simulink model "nounity"  (R2020a)
settings: Solver=FixedStepAuto  StartTime=0.0  StopTime=200  FixedStep=.005  RelTol=1e-3
undefined symbols (not defined in the file or in its folder): dMaxX, dMaxY, dMinX, dMinY, dSeedX, dSeedY, dts, waPhi, waPsi, waTheta, waX, waY, waZ, wfPhi, wfPsi, wfTheta, wfX, wfY, wfZ, wpPhi, wpPsi, wpTheta, wpX, wpY, wpZ
libraries: sharedutil x1
settings Model: Creator=Lamarre  LastModifiedBy=Lamarre

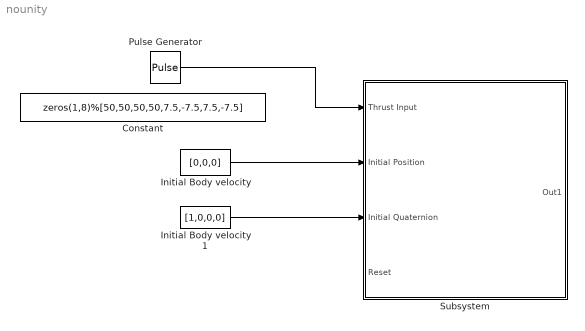
== system nounity ==
  Constant : Constant  Value=zeros(1,8)%[50,50,50,50,7.5,-7.5,7.5,-7.5]
  "Initial Body velocity " : Constant  Value=[0,0,0]
  Initial Body velocity 1 : Constant  Value=[1,0,0,0]
  Pulse Generator : DiscretePulseGenerator  PulseType=Time based  Amplitude=20  Period=10  PulseWidth=50
  Subsystem : Subsystem  InitFcn=|
      | % Initialiser le seed du random
      | rng shuffle
      | 
      | % Retrouver le paramètre de AUV8
      | cf = ConfigAUV8();
      | 
      | % Constante pour bloc areospace
      | %     I=cf.I;
      | %     mass=cf.mass;
      | 
      | % Perturbations des vages
      |     %Vages X
      |     waX=2;          % Amplitude
      |     wfX=pi/2;         % Frequence
      |     wpX=0;          % Phase
      |     %Vages Y
      |     waY=3;          % Amplitude
      |     wfY=pi/2;         % Frequence
      |     wpY=pi/2;       % Phase
      |     %Vages Z
      |     waZ= 4;         % Amplitude
      |     wfZ=pi/2;         % Frequence
      |     wpZ=pi;         % Phase
      |     %Vages RX (Roll)
      |     waPhi= 3;      % Amplitude
      |     wfPhi= pi/2;      % Frequence
      |     wpPhi=0;        % Phase
      |     %Vages Ry (Pitch)
      |     waTheta=3;    % Amplitude
      |     wfTheta=pi/2;     % Frequence
      |     wpTheta=pi/2;   % Phase
      |     %Vages Rz (Yaw)
      |     waPsi=3;       % Amplitude
      |     wfPsi=pi/2;       % Frequence
      |     wpPsi=pi;       % Phase
      |     
      | % Perturbation Drift
      | 
      |     dts=5; % Temp d'échantillionage des perturbation
      |     
      |     % Perturbation x
      |     dMinX=-1*rand(); % Valeur minimum x
      |     dMaxX=1*rand();  % Valeur maximum x
      |     dSeedX=round(rand*10);
      |     
      |     % Perturbation y
      |     dMinY=-3*rand(); % Valeur minimum  y
      |     dMaxY=3*rand();  % Valeur maximumx y
      |     dSeedY=round(rand*10);
  wires:
  "Initial Body velocity "/1 -> Subsystem/2(Initial Position)
  Initial Body velocity 1/1 -> Subsystem/3(Initial Quaternion)
  Pulse Generator/1 -> Subsystem/1(Thrust Input)

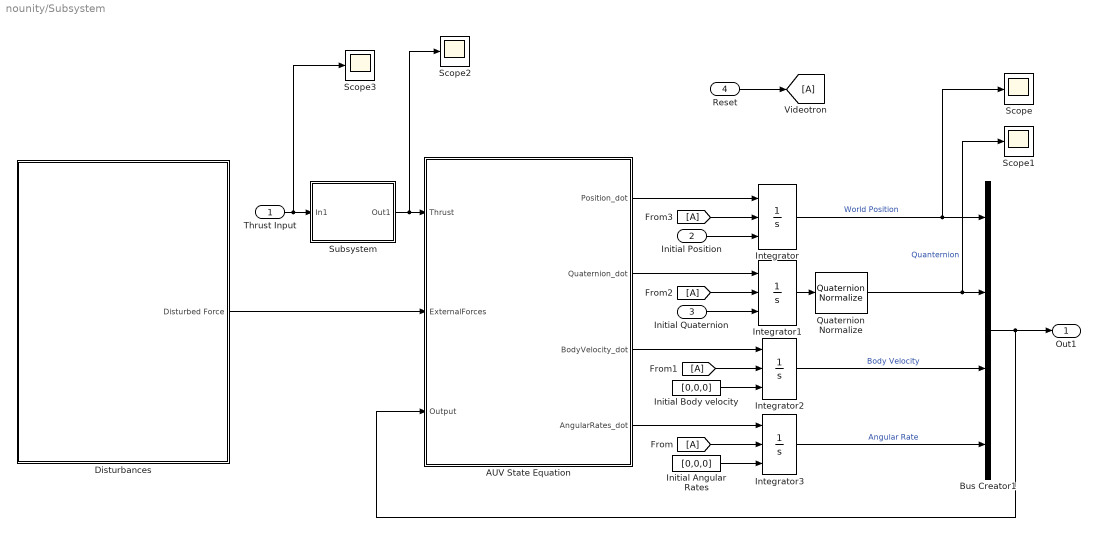
== system nounity/Subsystem ==
  Thrust Input : Inport
  Initial Position : Inport  Port=2
  Initial Quaternion : Inport  Port=3
  Reset : Inport  Port=4
  AUV State Equation : MATLAB Function  TreatAsAtomicUnit=on  SystemSampleTime=.005
  Bus Creator1 : BusCreator  Inputs=4
  Disturbances : Subsystem
  Initial Angular Rates : Constant  Value=[0,0,0]
  "Initial Body velocity " : Constant  Value=[0,0,0]
  Integrator : Integrator  ExternalReset=rising  InitialConditionSource=external  InitialCondition=[0,0,1]
  Integrator1 : Integrator  ExternalReset=rising  InitialConditionSource=external  InitialCondition=[1,0,0,0]
  Integrator2 : Integrator  ExternalReset=rising  InitialConditionSource=external  InitialCondition=[0,0,0]
  Integrator3 : Integrator  ExternalReset=rising  InitialConditionSource=external  InitialCondition=[0,0,0]
  Quaternion Normalize : sharedutil/Quaternion Normalize  aMode=aMode
      settings: SourceProductBaseCode=AE,PW,MT,VE,VP
  Scope{,1..3} (4 alike) : Scope
  Subsystem : Subsystem
  Out1 : Outport
  wires:
  "Initial Body velocity "/1 -> Integrator2/3
  Integrator1/1 -> Quaternion Normalize/1
  AUV State Equation/2(Quaternion_dot) -> Integrator1/1
  Integrator/1 -> Scope/1, Bus Creator1/1  "World Position"
  Integrator2/1 -> Bus Creator1/3  "Body Velocity"
  AUV State Equation/1(Position_dot) -> Integrator/1
  Initial Angular Rates/1 -> Integrator3/3
  Bus Creator1/1 -> Out1/1, AUV State Equation/3(Output)
  AUV State Equation/4(AngularRates_dot) -> Integrator3/1
  Quaternion Normalize/1 -> Scope1/1, Bus Creator1/2  "Quanternion"
  Integrator3/1 -> Bus Creator1/4  "Angular Rate"
  Initial Quaternion/1 -> Integrator1/3
  AUV State Equation/3(BodyVelocity_dot) -> Integrator2/1
  [A] -> Integrator3/2
  [A] -> Integrator2/2
  [A] -> Integrator1/2
  [A] -> Integrator/2
  Initial Position/1 -> Integrator/3
  Reset/1 -> [A]
  Disturbances/1(Disturbed Force) -> AUV State Equation/2(ExternalForces)
  Thrust Input/1 -> Scope3/1, Subsystem/1(In1)
  Subsystem/1(Out1) -> Scope2/1, AUV State Equation/1(Thrust)

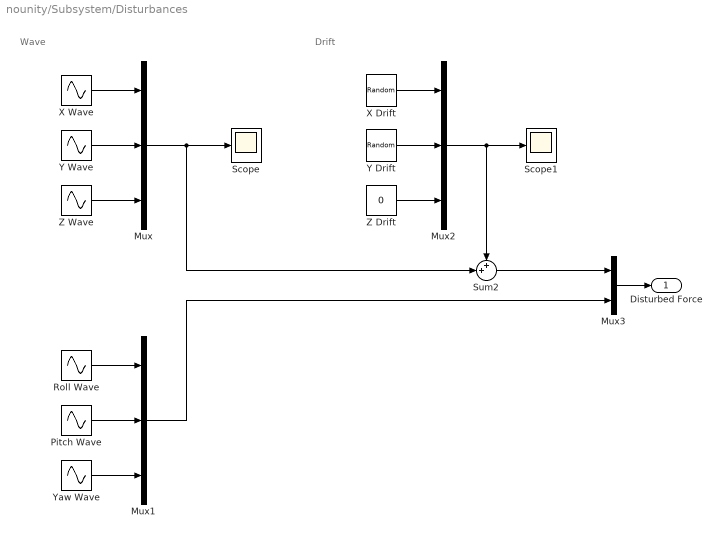
== system nounity/Subsystem/Disturbances ==
  note: Wave
  note: Drift
  Mux : Mux  Inputs=3
  Mux1 : Mux  Inputs=3
  Mux2 : Mux  Inputs=3
  Mux3 : Mux  Inputs=2
  Pitch Wave : Sin  Amplitude=waTheta  Frequency=wfTheta  Phase=wpTheta  SampleTime=0
  Roll Wave : Sin  Amplitude=waPhi  Frequency=wfPhi  Phase=wpPhi  SampleTime=0
  Scope : Scope
  Scope1 : Scope
  Sum2 : Sum  Inputs=++|
  X Drift : UniformRandomNumber  Minimum=dMinX  Maximum=dMaxX  Seed=dSeedX  SampleTime=dts
  X Wave : Sin  Amplitude=waX  Frequency=wfX  Phase=wpX  SampleTime=0
  Y Drift : UniformRandomNumber  Minimum=dMinY  Maximum=dMaxY  Seed=dSeedY  SampleTime=dts
  Y Wave : Sin  Amplitude=waY  Frequency=wfY  Phase=wpY  SampleTime=0
  Yaw Wave : Sin  Amplitude=waPsi  Frequency=wfPsi  Phase=wpPsi  SampleTime=0
  Z Drift : Constant  Value=0
  Z Wave : Sin  Amplitude=waZ  Frequency=wfZ  Phase=wpZ  SampleTime=0
  Disturbed Force : Outport
  wires:
  Z Drift/1 -> Mux2/3
  Mux/1 -> Scope/1, Sum2/2
  Y Drift/1 -> Mux2/2
  X Drift/1 -> Mux2/1
  Mux2/1 -> Sum2/1, Scope1/1
  Mux1/1 -> Mux3/2
  Yaw Wave/1 -> Mux1/3
  Roll Wave/1 -> Mux1/1
  Pitch Wave/1 -> Mux1/2
  Z Wave/1 -> Mux/3
  Y Wave/1 -> Mux/2
  X Wave/1 -> Mux/1
  Sum2/1 -> Mux3/1
  Mux3/1 -> Disturbed Force/1

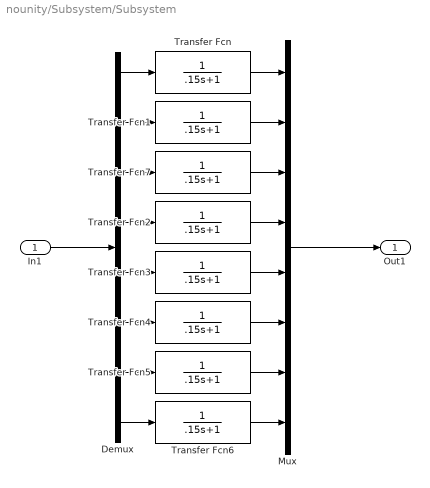
== system nounity/Subsystem/Subsystem ==
  In1 : Inport
  Demux : Demux  Outputs=8
  Mux : Mux  Inputs=8
  Transfer Fcn{,1..7} (8 alike) : TransferFcn  Denominator=[ .15 1]
  Out1 : Outport
  wires:
  In1/1 -> Demux/1
  Demux/1 -> Transfer Fcn/1
  Demux/2 -> Transfer Fcn1/1
  Demux/8 -> Transfer Fcn6/1
  Demux/7 -> Transfer Fcn5/1
  Demux/6 -> Transfer Fcn4/1
  Demux/5 -> Transfer Fcn3/1
  Demux/4 -> Transfer Fcn2/1
  Demux/3 -> Transfer Fcn7/1
  Transfer Fcn/1 -> Mux/1
  Transfer Fcn1/1 -> Mux/2
  Transfer Fcn7/1 -> Mux/3
  Transfer Fcn2/1 -> Mux/4
  Transfer Fcn3/1 -> Mux/5
  Transfer Fcn4/1 -> Mux/6
  Transfer Fcn5/1 -> Mux/7
  Transfer Fcn6/1 -> Mux/8
  Mux/1 -> Out1/1

== matlab function nounity/Subsystem/AUV State Equation ==
  data: Thrust input; ExternalForces input; Output input; Position_dot output size=3; Quaternion_dot output size=4; BodyVelocity_dot output size=3; AngularRates_dot output size=3
function [Position_dot,Quaternion_dot,BodyVelocity_dot, AngularRates_dot] = AUVStateEquation(Thrust,ExternalForces,Output)

Dynamics=AUVFossenSimFcn(Output,ExternalForces,Thrust);

Position_dot=Dynamics(1:3);
Quaternion_dot = Dynamics(4:7);
BodyVelocity_dot= Dynamics(8:10);
AngularRates_dot = Dynamics(11:13);
